simulink model "test"  (R2019b)
settings: Solver=VariableStepAuto  StartTime=0.0  StopTime=2.0  RelTol=1e-3
values from neighbouring files (symbols this model uses):
  abc = "abc"    [just_try_map.m]    (also in just_try_python.m = "abcd[sd]"; manual_env_for_test_slx.m = 0)
  Sample_time = 0.1    [main.m]    (also in manual_env_for_test_slx.m; test_tool_initialize.m)
settings Model: Creator=yangy  LastModifiedBy=yangy
settings DataIOCC: ExternalInput=ds.getElement(1),ds.getElement(2),ds.getElement(3)  LoadExternalInput=on

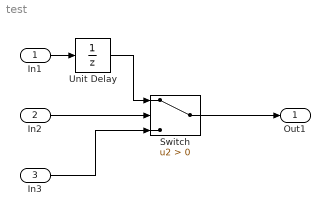
== system test ==
  In1 : Inport
  In2 : Inport  Port=2
  In3 : Inport  Port=3
  Switch : Switch  Criteria=u2 > Threshold
  Unit Delay : UnitDelay  InitialCondition=abc  SampleTime=Sample_time  HasFrameUpgradeWarning=on
  Out1 : Outport
  wires:
  In2/1 -> Switch/2
  In3/1 -> Switch/3
  Switch/1 -> Out1/1
  In1/1 -> Unit Delay/1
  Unit Delay/1 -> Switch/1
